simulink model "ProgettoLQplusKalman"  (R2021a)
settings: Solver=VariableStepAuto  StartTime=0.0  StopTime=30  RelTol=1e-3
undefined symbols (not defined in the file): A, AobsK, B, BobsK, CobsK, DobsK, K, Qt, Rt
libraries: simulink x3
settings Model: Creator=a15le  LastModifiedBy=a15le

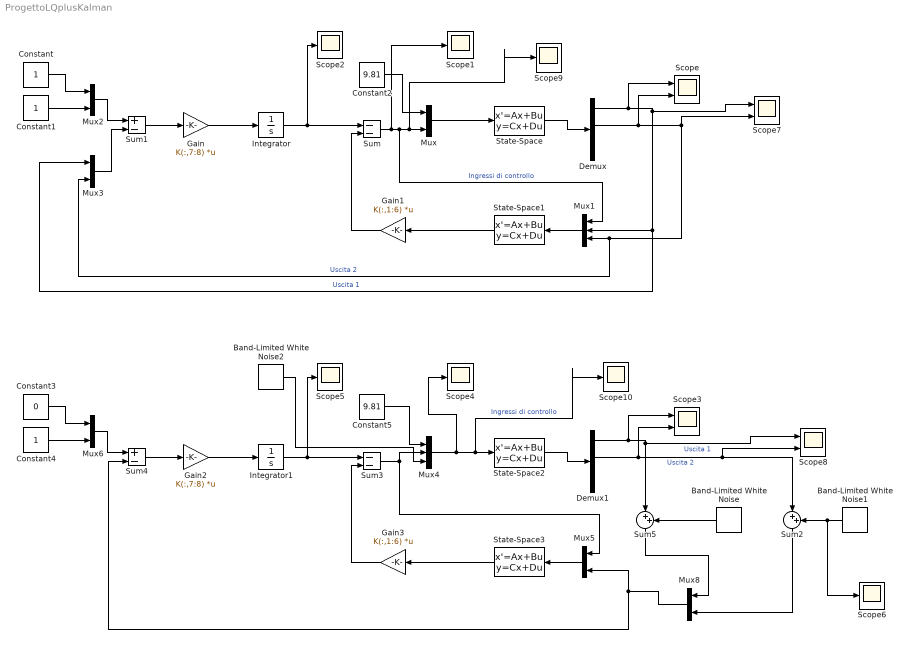
== system ProgettoLQplusKalman ==
  Band-Limited White Noise : simulink/Sources/Band-Limited White Noise  Cov=diag(Rt)*1e-3  Ts=1e-3  seed=[23341]
  Band-Limited White Noise1 : simulink/Sources/Band-Limited White Noise  Cov=diag(Rt)*1e-3  Ts=1e-3  seed=[23341]
  Band-Limited White Noise2 : simulink/Sources/Band-Limited White Noise  Cov=diag(Qt)*1e-3  Ts=1e-3  seed=[23341]
  Constant : Constant
  Constant1 : Constant
  Constant2 : Constant  Value=9.81
  Constant3 : Constant  Value=0
  Constant4 : Constant
  Constant5 : Constant  Value=9.81
  Demux : Demux  Outputs=6
  Demux1 : Demux  Outputs=6
  Gain : Gain  Gain=K(:,7:8)  Multiplication=Matrix(K*u)
  Gain1 : Gain  Gain=K(:,1:6)  Multiplication=Matrix(K*u)
  Gain2 : Gain  Gain=K(:,7:8)  Multiplication=Matrix(K*u)
  Gain3 : Gain  Gain=K(:,1:6)  Multiplication=Matrix(K*u)
  Integrator : Integrator
  Integrator1 : Integrator
  Mux{,2..3,5..6,8} (6 alike) : Mux  Inputs=2
  Mux1 : Mux  Inputs=3
  Mux4 : Mux  Inputs=3
  Scope{,3,7..8} (4 alike) : Scope  NumInputPorts=2
  Scope{1..2,4..6,9..10} (7 alike) : Scope
  State-Space : StateSpace  A=A  B=B  C=eye(6)  D=zeros(6,3)  InitialCondition=0
  State-Space1 : StateSpace  A=AobsK  B=BobsK  C=CobsK  D=DobsK  InitialCondition=0
  State-Space2 : StateSpace  A=A  B=[B eye(6)]  C=eye(6)  D=zeros(6,9)  InitialCondition=0
  State-Space3 : StateSpace  A=AobsK  B=BobsK  C=CobsK  D=DobsK  InitialCondition=0
  Sum : Sum  Inputs=--
  Sum1 : Sum  Inputs=+-
  Sum2 : Sum  Inputs=|++
  Sum3 : Sum  Inputs=--
  Sum4 : Sum  Inputs=+-
  Sum5 : Sum  Inputs=|++
  wires:
  State-Space/1 -> Demux/1
  Mux/1 -> State-Space/1
  Sum/1 -> Scope1/1, Mux1/1, Scope9/1, Mux/2  "Ingressi di controllo"
  Gain1/1 -> Sum/2
  Integrator/1 -> Scope2/1, Sum/1
  Gain/1 -> Integrator/1
  Constant/1 -> Mux2/1
  Constant1/1 -> Mux2/2
  Mux2/1 -> Sum1/1
  Mux1/1 -> State-Space1/1
  State-Space1/1 -> Gain1/1
  Sum1/1 -> Gain/1
  Demux/3 -> Scope/2, Mux3/2, Mux1/3, Scope7/2  "Uscita 2"
  Mux3/1 -> Sum1/2
  Demux/1 -> Scope7/1, Mux3/1, Mux1/2, Scope/1  "Uscita 1"
  Constant2/1 -> Mux/1
  Gain2/1 -> Integrator1/1
  State-Space2/1 -> Demux1/1
  Constant4/1 -> Mux6/2
  Mux5/1 -> State-Space3/1
  Gain3/1 -> Sum3/2
  Integrator1/1 -> Scope5/1, Sum3/1
  Band-Limited White Noise2/1 -> Mux4/3
  Band-Limited White Noise/1 -> Sum5/2
  State-Space3/1 -> Gain3/1
  Sum3/1 -> Mux4/2, Mux5/1
  Sum4/1 -> Gain2/1
  Constant3/1 -> Mux6/1
  Mux6/1 -> Sum4/1
  Sum5/1 -> Mux8/1
  Mux8/1 -> Mux5/2, Sum4/2
  Constant5/1 -> Mux4/1
  Band-Limited White Noise1/1 -> Scope6/1, Sum2/2
  Sum2/1 -> Mux8/2
  Demux1/1 -> Scope8/1, Sum5/1, Scope3/1  "Uscita 1"
  Demux1/3 -> Scope8/2, Sum2/1, Scope3/2  "Uscita 2"
  Mux4/1 -> Scope4/1, Scope10/1, State-Space2/1  "Ingressi di controllo"
